simulink model "TCAF_WHOLESIM"  (R2022a)
settings: Solver=ode4  StartTime=0.0  StopTime=150  FixedStep=0.01  RelTol=1e-3  EnableMultiTasking=on
PreLoadFcn:
  | listing = dir;
  | if (contains([listing .name], 'TPF')) && (contains([listing .name], 'MAP'))
  |     addpath('./TCAF', './TRN', './FTG', './DYN', './FLCC', './GPS', './RALT', './INS', './MAP');
  | elseif (contains([listing .name], 'TCAF_WHOLESIM.slx'))
  |     addpath('./TCAF', './TRN', './FTG', '../DYN', '../FLCC', '../GPS', '../RALT', '../INS', '../MAP');
  | else
  | 
  | end
  | addpath('C:\Users\ASCL\Documents\GitHub\DTNS\MAP\MAP_DB');
  | 
  | load('BUS_STRUCTURE_DYN.mat');
  | load('BUS_STRUCTURE_FLCC.mat');
  | load('BUS_STRUCTURE_RALT.mat');
  | load('BUS_STRUCTURE_INS.mat');
  | load('BUS_STRUCTURE_GPS.mat');
  | load('BusStructureTRN.mat');
  | load('BusStructureWTPG.mat');
  | load('BusStructureDTF.mat');
  | load('BusStructureGCAWS.mat');
  | FTG_initState;
InitFcn:
  | listing = dir;
  | if (contains([listing .name], 'TPF')) && (contains([listing .name], 'MAP'))
  |     addpath('./TCAF', './TRN', './FTG', './DYN', './FLCC', './GPS', './RALT', './INS', './MAP');
  | elseif (contains([listing .name], 'TCAF_WHOLESIM.slx'))
  |     addpath('./TCAF', './TRN', './FTG', '../DYN', '../FLCC', '../GPS', '../RALT', '../INS', '../MAP');
  | else
  | 
  | end
  | 
  | load('BUS_STRUCTURE_DYN.mat');
  | load('BUS_STRUCTURE_FLCC.mat');
  | load('BUS_STRUCTURE_RALT.mat');
  | load('BUS_STRUCTURE_INS.mat');
  | load('BUS_STRUCTURE_GPS.mat');
  | load('BusStructureTRN.mat');
  | load('BusStructureWTPG.mat');
  | load('BusStructureDTF.mat');
  | load('BusStructureGCAWS.mat');
  | FTG_initState;
  | 
  | clear 'logsout'
libraries: aerolibconvert2 x14, simulink_extras x5
(part 2 of 2)

== matlab function TCAF_WHOLESIM/VisualizeWTPOnly ==
  data: wtp input; predictedTraj input
function VisualizeWTPOnly(wtp, predictedTraj)
%VisualizeWTPOnly
% 
persistent fHandle subPlot1 subPlot2 tSpanWCP tSpanPT count map ARCSEC2DEG mapSurf predBound yAxisMax

acXY = zeros(2,27);
heading = 0;

% Initialize Figure Handle
if isempty(fHandle)
    fHandle = figure('WindowStyle', 'docked');
end

% Divide and Initailize the Figure
if isempty(subPlot1)
    set(0, 'CurrentFigure', fHandle);
%     subPlot1 = subplot(5, 1, 1:4, 'position', [0.05 0.525 0.9 0.425]);
    subPlot1 = subplot(1, 4, 1:2);
    axis equal;
    colormap(fliplr(hsv));
    view(0, 90);
    set(gca, 'Color', [0.3, 0.3, 0.3]);
    xlabel('Longitude [deg]');
    ylabel('Latitude [deg]');
    hold off;
end

% Divide and Initailize the Figure
if isempty(subPlot2)
%     subPlot2 = subplot(5, 1, 5, 'position', [0.1 0.05 0.8 0.425]);
    subPlot2 = subplot(1, 4, 3:4);
    hold on;
    grid minor;
    xlabel('Time [sec]');
    ylabel('Height [m]');
    axis([-0.5, 20, 0, 2000]);
    hold off;
end

% Initialize tSpanWCP
if isempty(tSpanWCP)
    tSpanWCP = 0:0.5:((length(wtp)-1)*0.5);
end

% Initialize tSpanPT
if isempty(tSpanPT)
    tSpanPT = 0:0.25:((size(predictedTraj, 1)-1)*0.25);
end

% Initialize count
if isempty(count)
    count = 0;    
end

% Initialize yAxisMax
if isempty(yAxisMax) 
    yAxisMax = 2000;
end
% Initialize ARCSEC2DEG
if isempty(ARCSEC2DEG)
    ARCSEC2DEG = (0.000277777777777777);
end

% Initialize map
if isempty(map)
    map = ones(150, 150, 3);

    % Current A/C Position
    latTrue = predictedTraj(1, 1, 1);
    lonTrue = predictedTraj(1, 1, 2);
    
    % Flooring to neighboring Map Grid
    latTrun = floor(latTrue/(3*ARCSEC2DEG)) * (3*ARCSEC2DEG);
    lonTrun = floor(lonTrue/(3*ARCSEC2DEG)) * (3*ARCSEC2DEG);
    
    mapSizeLat = size(map, 1);
    mapSizeLon = size(map, 2);
    % Update map data
    for ii = 1:size(map, 1)
    
        for jj = 1:size(map, 2)
            
            map(ii, jj, 1) = latTrun + (9*ARCSEC2DEG) * ((size(map, 1) - floor(mapSizeLat * 1.5)) + ii);
            map(ii, jj, 2) = lonTrun + (9*ARCSEC2DEG) * ((size(map, 2) - floor(mapSizeLon * 1.5)) + jj);
            
            map(ii, jj, 3) = ...
            coder.ceval('MAPGetTerrainHeight', map(ii, jj, 1), map(ii, jj, 2)); 
            if (ii == size(map, 1)) && (jj == size(map,2))
                map(ii, jj, 3) = 2000;
            end
            
        end
    
    end
    
end

% Initialize mapSurf: mapSurf plot handle
if isempty(mapSurf)
    set(0, 'CurrentFigure', fHandle);
    subplot(subPlot1);
    hold on;
    mapSurf = surf(map(:,:,2), map(:,:,1), map(:,:,3), 'FaceAlpha', 0.85);
    drawnow;
    hold off;
end

% Initialize predBound: predBound plot handle
if isempty(predBound)
    set(0, 'CurrentFigure', fHandle);
    subplot(subPlot1);
    hold on;
    predBound = plot3([predictedTraj(:,2,2); flipud(predictedTraj(:,3,2))], ...
        [predictedTraj(:,2,1); flipud(predictedTraj(:,3,1))], ...
        [predictedTraj(:,2,3); flipud(predictedTraj(:,3,3))], '-m', 'LineWidth', 3);
    hold off;
end


%%

% Limit & Reset count
if (count >= 250)
    count = 0;
end

% 5Hz Event
if rem(count, 5) == 0
    set(0, 'CurrentFigure', fHandle);
    subplot(subPlot1);
    hold on;
    
    % Current A/C Position
    latTrue = predictedTraj(1, 1, 1);
    lonTrue = predictedTraj(1, 1, 2);
    
    % Flooring to neighboring Map Grid
    latTrun = floor(latTrue/(3*ARCSEC2DEG)) * (3*ARCSEC2DEG);
    lonTrun = floor(lonTrue/(3*ARCSEC2DEG)) * (3*ARCSEC2DEG);
    
    mapSizeLat = size(map, 1);
    mapSizeLon = size(map, 2);
    if abs(latTrun-(map(1, 1, 1)+map(end, 1, 1))/2) >= 100*(3*ARCSEC2DEG) || abs(lonTrun-(map(1, 1, 2)+map(1, end, 2))/2) >= 100*(3*ARCSEC2DEG)
        % Update map data
        for ii = 1:size(map, 1)
            for jj = 1:size(map, 2)
                map(ii, jj, 1) = latTrun + (9*ARCSEC2DEG) * ((size(map, 1) - floor(mapSizeLat * 1.5)) + ii);
                map(ii, jj, 2) = lonTrun + (9*ARCSEC2DEG) * ((size(map, 2) - floor(mapSizeLon * 1.5)) + jj);
                map(ii, jj, 3) = ...
                coder.ceval('MAPGetTerrainHeight', map(ii, jj, 1), map(ii, jj, 2)); 
            end
        end
        
        set(mapSurf, 'XData', map(:,:,2), 'YData', map(:,:,1), 'ZData', map(:,:,3));
        drawnow;
    end
    
    % Draw Map
    axis([lonTrun - (3*ARCSEC2DEG)*60, lonTrun + (3*ARCSEC2DEG)*60, latTrun - (3*ARCSEC2DEG)*60, latTrun + (3*ARCSEC2DEG)*60]);
    drawnow;
    hold off;
    
end

% 2.5Hz Event
if rem(count, 5) == 0
    set(0, 'CurrentFigure', fHandle);
    subplot(subPlot1);
    
    hold on;
    latTrue = predictedTraj(1, 1, 1);
    lonTrue = predictedTraj(1, 1, 2);
    heading = getHeadingFromVector([latTrue, lonTrue], [predictedTraj(81, 1, 1), predictedTraj(81, 1, 2)]);
    acXY = drawAircraft( [lonTrue;latTrue], 4.5*ARCSEC2DEG, heading);
    plot3(acXY(1,:), acXY(2,:), predictedTraj(1, 1, 3)*ones(size(acXY(1,:))), '-r')
    
    set(predBound, 'XData', [predictedTraj(:,2,2); flipud(predictedTraj(:,3,2))], ...
    'YData', [predictedTraj(:,2,1); flipud(predictedTraj(:,3,1))], ...
    'ZData', [predictedTraj(:,2,3); flipud(predictedTraj(:,3,3))]+200);
    
    hold off;
    
    set(0, 'CurrentFigure', fHandle);
    subplot(subPlot2);
    
    nominalTerrain = zeros(size(predictedTraj, 1), 1);
    for nn = 1:size(predictedTraj(:,1,3), 1)
        nominalTerrain(nn) = coder.ceval('MAPGetTerrainHeight', predictedTraj(nn, 1, 1), predictedTraj(nn, 1, 2)); 
    end
    
    hold on;
    cla
    plot(tSpanPT, nominalTerrain, '-g', 'LineWidth', 5, 'DisplayName', 'Nominal Terrain');
    plot(tSpanWCP, wtp, '-b', 'LineWidth', 5, 'DisplayName', 'WCP');

    if (predictedTraj(1, 1, 3) > yAxisMax-300)
        axis([-0.5, 20, 0, predictedTraj(1, 1, 3) + 500]);
    elseif (predictedTraj(1, 1, 3) < 1800)
        axis([-0.5, 20, 0, 2000])
    end
    % axis([-1, 20, 300, 800]);
    drawnow;
    hold off; 
    
end

% Update count
count = count + 1;

end


function [acXY] = drawAircraft(centerXY, longLength, heading)
%DRAWAircraft
    % centerXY      (2x1)
    % longLength    (1) [deg]
    % heading       (1) [deg]
    
    acXY = zeros(2, 27);
    translate = ones(2, 27);
    translate(1,:) = translate(1,:) * centerXY(1); 
    translate(2,:) = translate(2,:) * centerXY(2); 
    
    refXY = [ 0, -2, -4, -6,-16,-16,-17,-17, -4, -4, -9,-10, -4,  0,  4, 10,  9,  4,  4, 17, 17, 16, 16,  6,  4,  2,  0;...
             25, 20,  8,  0, -7, -4, -4,-14,-14,-18,-23,-26,-25,-25,-25,-26,-23,-18,-14,-14, -4, -4, -7,  0,  8, 20, 25];
    
    acXY = refXY / 50 * longLength;
    
    rot = [cosd(-heading), -sind(-heading); sind(-heading), cosd(-heading)];
    
    acXY = rot * acXY + translate;
    
end

function [heading] = getHeadingFromVector(fromLatLon, toLatLon)
%GETHEADINGFROMVECTOR
    % fromLatLon (2x1) [deg]
    % toLatLon (2x1) [deg]
    
    dLon = toLatLon(2) - fromLatLon(2);
    
    y = sind(dLon) * cosd(toLatLon(1));
    x = cosd(fromLatLon(1)) * sind(toLatLon(1)) ...
        - sind(fromLatLon(1)) * cosd(toLatLon(1)) * cosd(dLon);
    
    heading = atan2d(y, x);
    heading = rem( heading + 360, 360);

end

== matlab function TCAF_WHOLESIM/ControlGCAWSInput ==
  data: inBus input Bus: GCAWSInput; GCAWWSInput output Bus: GCAWSInput
function GCAWWSInput = ControlGCAWSInput(inBus)
%ControlGCAWSInput
persistent time dt
if isempty(time)
    time = 0.0;
end
if isempty(dt)
    dt = 0.01;
end
% -------------------------------------------------------------------------
% CONTROL flag
CONTROL_ACTIVATED = true;

% Copy
GCAWWSInput = inBus;

if CONTROL_ACTIVATED
    % Default
    GCAWWSInput.selected        = SET_VALUE(GCAWWSInput.selected,       true, time, 0, inf);
    GCAWWSInput.paramSelected   = SET_VALUE(GCAWWSInput.paramSelected,  true, time, 0, inf);
    GCAWWSInput.reactionTime        = SET_VALUE(GCAWWSInput.reactionTime,       uint16(3), time, 0, inf);
    GCAWWSInput.rollRate            = SET_VALUE(GCAWWSInput.rollRate,           uint16(3), time, 0, inf);
    GCAWWSInput.gOnsetRate          = SET_VALUE(GCAWWSInput.gOnsetRate,         uint16(1), time, 0, inf);
    GCAWWSInput.pullUpG             = SET_VALUE(GCAWWSInput.pullUpG,            uint16(1), time, 0, inf);
    GCAWWSInput.maxFlightPathAngle  = SET_VALUE(GCAWWSInput.maxFlightPathAngle, uint16(1), time, 0, inf);
    GCAWWSInput.gsAvailable         = SET_VALUE(GCAWWSInput.gsAvailable, 5.0, time, 0, inf);
    GCAWWSInput.gsAvaliableValid    = SET_VALUE(GCAWWSInput.gsAvaliableValid, true, time, 0, inf);
    GCAWWSInput.swh                 = SET_VALUE(GCAWWSInput.swh, single(100), time, 0, inf);

    % Control
%     outBus.msd = SET_VALUE(outBus.msd, 500, time, 100, 50);
%     outBus.msd = SET_VALUE(outBus.msd, 500, time, 200, 50);

end

% Update Time
time = time + dt;
end

function out = SET_VALUE(in, value, curTime, triggerTime, duration)
out = in;
if (triggerTime <= curTime) && (curTime <= triggerTime+duration)
    out = value;
else
end
end

== matlab function TCAF_WHOLESIM/ControlTFInput ==
  data: inBus input Bus: DTFInput; DTFInput output Bus: DTFInput; RALTDatapumpPrev input
function DTFInput = ControlTFInput(inBus, RALTDatapumpPrev)
%ControlTFInput
persistent time dt
if isempty(time)
    time = 0.0;
end
if isempty(dt)
    dt = 0.01;
end
% -------------------------------------------------------------------------
% CONTROL flag
CONTROL_ACTIVATED = true;

% Copy
DTFInput = inBus;

if CONTROL_ACTIVATED
    % Default
    DTFInput.selected   = SET_VALUE(DTFInput.selected, true, time, 0, inf);
    DTFInput.rideQuality= SET_VALUE(DTFInput.rideQuality, uint16(3), time, 0, inf);
    DTFInput.msd        = SET_VALUE(DTFInput.msd, 500, time, 0, inf);
    DTFInput.raltValid  = SET_VALUE(DTFInput.raltValid, RALTDatapumpPrev.RadarAltitudeValid, time, 0, inf);
    DTFInput.raltAlt    = SET_VALUE(DTFInput.raltAlt, RALTDatapumpPrev.RadarAltitude, time, 0, inf);

    % Control
%     outBus.msd = SET_VALUE(outBus.msd, 500, time, 100, 50);
%     outBus.msd = SET_VALUE(outBus.msd, 500, time, 200, 50);

end

% Update Time
time = time + dt;
end

function out = SET_VALUE(in, value, curTime, triggerTime, duration)
out = in;
if (triggerTime <= curTime) && (curTime <= triggerTime+duration)
    out = value;
else
end
end

== matlab function TCAF_WHOLESIM/TRNDataProcess/Subsystem3/Flag_WoW ==
  data: time input; WeightOnWheels output
function WeightOnWheels  = fcn(time)

% WeightOnWheels
% False[0]_flight / True[1]_ground

% if time <= 30
if time < 0
    WeightOnWheels = boolean(true);
else
    WeightOnWheels = boolean(false);
end

end

== matlab function TCAF_WHOLESIM/TRNDataProcess/Subsystem3/MATLAB Function ==
  data: count input; count output
function count = fcn(count)

count = count + 0.04;

== matlab function TCAF_WHOLESIM/TRNDataProcess/Subsystem3/Subsystem1/MATLAB Function1 ==
  data: WoW input; time input; lat_bias output; lon_bias output
function [lat_bias,lon_bias] = fcn(WoW, time)
%% parameters
lat2m = 111000;
lon2m = 91170;
bias1 = 200;   % 500m
bias2 = 200;   % 500m


%%
% if time > 60
if time >= 0
    if WoW == 0                % 0_flight / 1_ground
        lat_bias = bias1/lat2m;
        lon_bias = bias2/lon2m;
    else
        lat_bias = 0;
        lon_bias = 0;
    end
else
    lat_bias = 0;
    lon_bias = 0;
end

== matlab function TCAF_WHOLESIM/TRNDataProcess/Subsystem3/Subsystem1/MATLAB Function3 ==
  data: u input; a output; b output
function [a,b]  = fcn(u)

% WeightOnWheels
if(u==1)
    a = boolean(true);
    b = boolean(true);
else
    a = boolean(false);
    b = boolean(false);
end

end

== matlab function TCAF_WHOLESIM/calcTerrainRoughness ==
  data: lat input; R output; lon input; hDEM output
function [R, hDEM] = calcTerrainRoughness(lat, lon)

lat2m = 110961.7060516;
lon2m = 89476.51124;

d_Lat = 90/lat2m; d_Lon = 90/lon2m;
d = 90;

hDEM = 0.0;
A=0.0; B=0.0; C=0.0; D=0.0; E=0.0; F=0.0; G=0.0; H=0.0; I=0.0; 

A = coder.ceval('MAPGetTerrainHeight', lat+d_Lat, lon-d_Lon);
B = coder.ceval('MAPGetTerrainHeight', lat+d_Lat, lon);
C = coder.ceval('MAPGetTerrainHeight', lat+d_Lat, lon+d_Lon);
D = coder.ceval('MAPGetTerrainHeight', lat, lon-d_Lon);
E = coder.ceval('MAPGetTerrainHeight', lat, lon);
F = coder.ceval('MAPGetTerrainHeight', lat, lon+d_Lon);
G = coder.ceval('MAPGetTerrainHeight', lat-d_Lat, lon-d_Lon);
H = coder.ceval('MAPGetTerrainHeight', lat-d_Lat, lon);
I = coder.ceval('MAPGetTerrainHeight', lat-d_Lat, lon+d_Lon);

SLP_CR=((C+F+I)-(A+D+G))/(6*d);
SLP_DR=((A+B+C)-(G+H+I))/(6*d);

mean_R=((mean(SLP_CR)-mean(SLP_DR))/2)^2;
std_R=((std(SLP_CR)^2)+(std(SLP_DR)^2))/2;

R=sqrt(mean_R+std_R)*100;

hDEM = E;

end
